simulink model "MBD_Prob5"  (R2020a)
settings: Solver=VariableStepAuto  StartTime=0.0  StopTime=10.0  RelTol=1e-3
model workspace (MAT data in the model file):
  C = 10
  R = 10
settings Model: Creator=Noel Varghese  LastModifiedBy=Noel Varghese

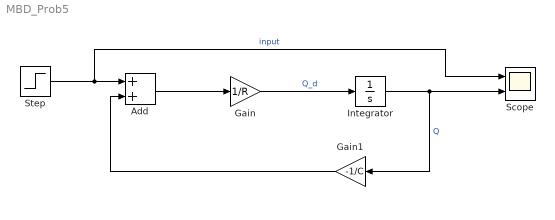
== system MBD_Prob5 ==
  Add : Sum
  Gain : Gain  Gain=1/R
  Gain1 : Gain  Gain=-1/C
  Integrator : Integrator
  Scope : Scope  NumInputPorts=2
  Step : Step  SampleTime=0
  wires:
  Gain/1 -> Integrator/1  "Q_d"
  Integrator/1 -> Gain1/1, Scope/2  "Q"
  Add/1 -> Gain/1
  Gain1/1 -> Add/2
  Step/1 -> Scope/1, Add/1  "input"
